simulink model "testpidPend"  (Simulink 6.0)
settings: Solver=ode45  StartTime=0  StopTime=10  MaxStep=0.5  RelTol=1e-3
libraries: simulink x2
settings Model: LastModifiedBy=jj
settings DataIOCC: LimitDataPoints=off
settings OptimizationCC: InlineInvariantSignals=off

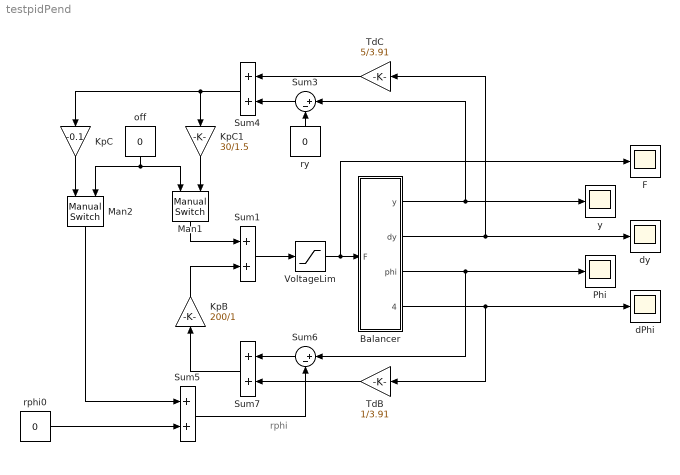
== system testpidPend ==
  note: rphi
  Balancer : Subsystem
  F : Scope
      settings: TimeRange=10  YMin=-15  YMax=10
  KpB : Gain  Orientation=up  Gain=200/1
  KpC : Gain  Orientation=down  Gain=-0.1
  KpC1 : Gain  Orientation=down  Gain=30/1.5
  Man1 : simulink/Signal Routing/Manual Switch  Orientation=down  sw=0  action=0
  Man2 : simulink/Signal Routing/Manual Switch  Orientation=down  sw=0  action=0
  Phi : Scope
      settings: TimeRange=10  YMin=-0.3  YMax=0.2  MaxDataPoints=50000
  Sum1 : Sum
  Sum3 : Sum  Orientation=left  Inputs=|+-
  Sum4 : Sum  Orientation=left
  Sum5 : Sum
  Sum6 : Sum  Orientation=left  Inputs=|+-
  Sum7 : Sum  Orientation=left
  TdB : Gain  Orientation=left  Gain=1/3.91
  TdC : Gain  Orientation=left  Gain=5/3.91
  VoltageLim : Saturate  UpperLimit=13  LowerLimit=-13
  dPhi : Scope
      settings: TimeRange=50  YMin=0  YMax=1.5  SaveName=ScopeData3  MaxDataPoints=50000
  dy : Scope
      settings: TimeRange=1000  YMin=-1  YMax=2  SaveName=ScopeData5
  off : Constant  Orientation=down  Value=0
  rphi0 : Constant  Value=0
  ry : Constant  Orientation=up  Value=0
  y : Scope
      settings: TimeRange=10  YMin=-0.8  YMax=0.6  SaveName=ScopeData4
  wires:
  Balancer/1(y) -> y/1, Sum3/1
  Balancer/2(dy) -> dy/1, TdC/1
  Sum4/1 -> KpC1/1, KpC/1
  Balancer/4(dphi) -> dPhi/1, TdB/1
  Sum1/1 -> VoltageLim/1
  VoltageLim/1 -> F/1, Balancer/1(F)
  Balancer/3(phi) -> Phi/1, Sum6/1
  TdC/1 -> Sum4/1
  KpB/1 -> Sum1/2
  Sum3/1 -> Sum4/2
  ry/1 -> Sum3/2
  Sum6/1 -> Sum7/1
  TdB/1 -> Sum7/2
  Sum7/1 -> KpB/1
  rphi0/1 -> Sum5/2
  Sum5/1 -> Sum6/2
  Man1/1 -> Sum1/1
  KpC1/1 -> Man1/2
  off/1 -> Man1/1, Man2/2
  KpC/1 -> Man2/1
  Man2/1 -> Sum5/1

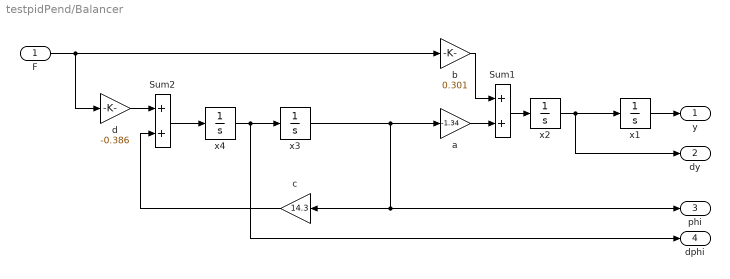
== system testpidPend/Balancer ==
  F : Inport  Port=1  LatchInput=off
  Sum1 : Sum
  Sum2 : Sum
  a : Gain  Gain=-1.34
  b : Gain  Gain=0.301
  c : Gain  Orientation=left  Gain=14.3
  d : Gain  Gain=-0.386
  x1 : Integrator  InitialCondition=0.525
  x2 : Integrator
  x3 : Integrator  InitialCondition=-0.22  UpperSaturationLimit=0.22  LowerSaturationLimit=-0.22
  x4 : Integrator
  y : Outport
  dy : Outport  Port=2
  phi : Outport  Port=3
  dphi : Outport  Port=4
  wires:
  Sum1/1 -> x2/1
  Sum2/1 -> x4/1
  x2/1 -> x1/1, dy/1
  a/1 -> Sum1/2
  x4/1 -> x3/1, dphi/1
  c/1 -> Sum2/2
  b/1 -> Sum1/1
  F/1 -> d/1, b/1
  d/1 -> Sum2/1
  x1/1 -> y/1
  x3/1 -> a/1, c/1, phi/1
